simulink model "tailsitter_simulation_main_copy"  (R2021a)
settings: Solver=VariableStepAuto  StartTime=0.0  StopTime=tf  RelTol=1e-3
values from neighbouring files (symbols this model uses):
  b = 0.6    [linear_dynamics_hover.m]    (also in nonlinear_dynamics_eq.m; simulink_setup.m; tailsitter.m; tailsitter_sym.m)
  c_bar = 0.142    [linear_dynamics_hover.m]    (also in nonlinear_dynamics_eq.m; simulink_setup.m; tailsitter.m; tailsitter_sym.m)
  CD_f = 0.000762    [linear_dynamics_hover.m]    (also in nonlinear_dynamics_eq.m; simulink_setup.m; tailsitter.m; tailsitter_sym.m)
  CL_0 = 0    [linear_dynamics_hover.m]    (also in nonlinear_dynamics_eq.m; simulink_setup.m; tailsitter.m; tailsitter_sym.m)
  CL_f = 0.036    [linear_dynamics_hover.m]    (also in nonlinear_dynamics_eq.m; simulink_setup.m; tailsitter.m; tailsitter_sym.m)
  Cl_f = 0.0057    [linear_dynamics_hover.m]    (also in nonlinear_dynamics_eq.m; simulink_setup.m; tailsitter.m; tailsitter_sym.m)
  Cm_0 = 0    [linear_dynamics_hover.m]    (also in nonlinear_dynamics_eq.m; simulink_setup.m; tailsitter.m; tailsitter_sym.m)
  Cm_f = -0.0102    [linear_dynamics_hover.m]    (also in nonlinear_dynamics_eq.m; simulink_setup.m; tailsitter.m; tailsitter_sym.m)
  CP = 0.01    [linear_dynamics_hover.m]    (also in nonlinear_dynamics_eq.m; simulink_setup.m; tailsitter.m; tailsitter_sym.m)
  CT = 0.05    [linear_dynamics_hover.m]    (also in nonlinear_dynamics_eq.m; simulink_setup.m; tailsitter.m; tailsitter_sym.m)
  D = 0.12    [linear_dynamics_hover.m]    (also in nonlinear_dynamics_eq.m; simulink_setup.m; tailsitter.m; tailsitter_sym.m)
  dt = 0.005    [simulink_setup.m]    (also in tailsitter_test.m)
  g = 9.81    [linear_dynamics_hover.m]    (also in nonlinear_dynamics_eq.m; simulink_setup.m; tailsitter.m; tailsitter_sym.m)
  J = [Jxx 0 -Jxz; 0 Jyy 0; -Jxz 0 Jzz]    [linear_dynamics_hover.m]    (also in nonlinear_dynamics_eq.m; simulink_setup.m; tailsitter.m; tailsitter_sym.m)
  Kd = 0.01    [simulink_setup.m]
  Kp = 1    [simulink_setup.m]    (also in tailsitter_test.m = 10)
  Kpi = 10    [simulink_setup.m]    (also in tailsitter_test.m = 100)
  Kq = 1    [simulink_setup.m]    (also in tailsitter_test.m = 10)
  Kqi = 20    [simulink_setup.m]    (also in tailsitter_test.m = 50)
  Kr = 5    [simulink_setup.m]    (also in tailsitter_test.m = 10)
  Kri = 20    [simulink_setup.m]    (also in tailsitter_test.m = 5)
  Kt = -5    [simulink_setup.m]    (also in tailsitter_test.m)
  Kti = -100    [simulink_setup.m]    (also in tailsitter_test.m)
  m = 0.3    [linear_dynamics_hover.m]    (also in nonlinear_dynamics_eq.m; simulink_setup.m; tailsitter.m; tailsitter_sym.m)
  M_flap = [-1 1; -1 -1]    [simulink_setup.m]    (also in tailsitter_test.m)
  M_motor = [1 1; 1 -1]    [simulink_setup.m]    (also in tailsitter_test.m)
  motor_eq = xeq(end)    [simulink_setup.m]
  prop_arm = 0.15    [linear_dynamics_hover.m]    (also in nonlinear_dynamics_eq.m; simulink_setup.m; tailsitter.m; tailsitter_sym.m)
  rho = 1.225    [linear_dynamics_hover.m]    (also in nonlinear_dynamics_eq.m; simulink_setup.m; tailsitter.m; tailsitter_sym.m)
  S_w = S_w/3    (= 0.0276)    [linear_dynamics_hover.m]    (also in nonlinear_dynamics_eq.m; simulink_setup.m = 0.0828; tailsitter.m = 0.0828; tailsitter_sym.m)
libraries: sharedtransform x6, pid_lib x4, vrlib x3, simulink x2, aerolibutil x2, simulink_extras x1, sharedutil x1
settings Model: PacingRate=0.032000  Creator=Owner  LastModifiedBy=Owner

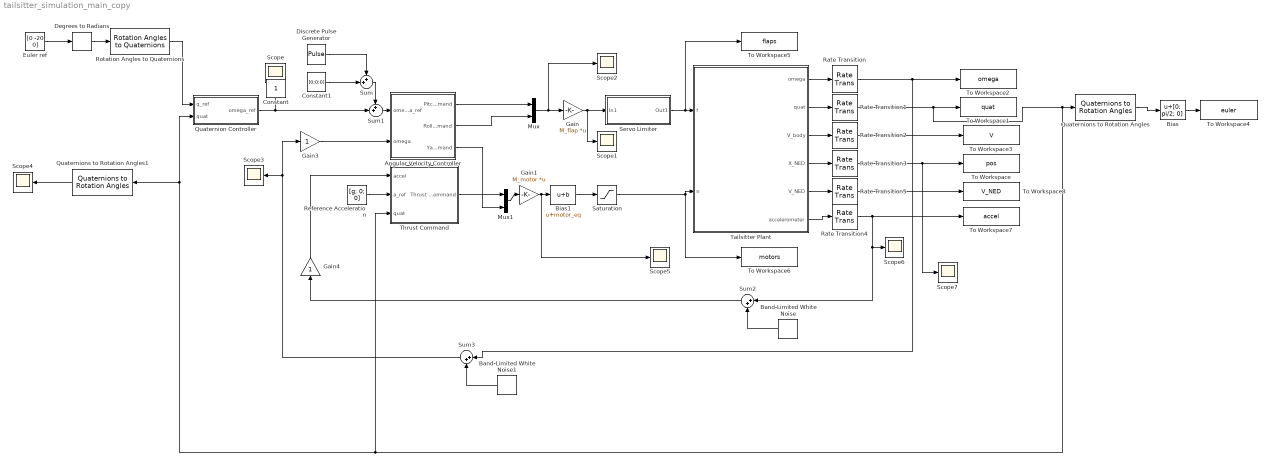
== system tailsitter_simulation_main_copy ==
  Angular Velocity Controller : Subsystem
  Band-Limited White Noise : simulink/Sources/Band-Limited White Noise  Cov=0.01  Ts=dt  seed=[23341]
  Band-Limited White Noise1 : simulink/Sources/Band-Limited White Noise  Cov=0.0001  Ts=dt  seed=[23341]
  Bias : Bias  Bias=[0; pi/2; 0]
  Bias1 : Bias  Bias=motor_eq
  Constant1 : Constant  Value=[0;0;0]  SampleTime=dt
  Degrees to Radians : simulink_extras/Transformations/Degrees to Radians
  Discrete Pulse Generator : DiscretePulseGenerator  Amplitude=0  Period=100000  PulseWidth=20  PhaseDelay=100  SampleTime=dt
  Euler ref : Constant  Value=[0 -20 0]  SampleTime=dt
  Gain : Gain  Gain=M_flap  Multiplication=Matrix(K*u)
  Gain1 : Gain  Gain=M_motor  Multiplication=Matrix(K*u)
  Gain3 : Gain
  Gain4 : Gain
  Mux : Mux  Inputs=2
  Mux1 : Mux  Inputs=2
  Quaternion Controller : Subsystem
  Quaternions to Rotation Angles : sharedtransform/Quaternions to Rotation Angles  rotationOrder=ZYX  aMode=aMode
      settings: SourceProductBaseCode=AE,PW,DR,MT,UV,VE
  Quaternions to Rotation Angles1 : sharedtransform/Quaternions to Rotation Angles  rotationOrder=ZYX  aMode=aMode
      settings: SourceProductBaseCode=AE,PW,DR,MT,UV,VE
  Rate Transition{,1..3,5} (5 alike) : RateTransition  OutPortSampleTime=dt
  Rate Transition4 : RateTransition  OutPortSampleTime=0.005
  Reference Acceleration : Constant  Value=[g; 0; 0]  SampleTime=dt
  Rotation Angles to Quaternions : sharedtransform/Rotation Angles to Quaternions  rotationOrder=ZYX  aMode=aMode
      settings: SourceProductBaseCode=AE,PW,DR,MT,UV,VE
  Saturation : Saturate  UpperLimit=500  LowerLimit=0
  Scope{,1..7} (8 alike) : Scope
  Servo Limiter : Subsystem
  Sum : Sum  Inputs=++|
  Sum1 : Sum  Inputs=++|
  Sum2 : Sum  Inputs=|++
  Sum3 : Sum  Inputs=|++
  Tailsitter Plant : Subsystem
  Thrust Command : Subsystem
  To Workspace : ToWorkspace  VariableName=pos  SampleTime=-1
  To Workspace1 : ToWorkspace  VariableName=quat  SampleTime=-1
  To Workspace2 : ToWorkspace  VariableName=omega  SampleTime=-1
  To Workspace3 : ToWorkspace  VariableName=V  SampleTime=-1
  To Workspace4 : ToWorkspace  VariableName=euler  SampleTime=-1
  To Workspace5 : ToWorkspace  VariableName=flaps  SampleTime=-1
  To Workspace6 : ToWorkspace  VariableName=motors  SampleTime=-1
  To Workspace7 : ToWorkspace  VariableName=accel  SampleTime=-1
  To Workspace8 : ToWorkspace  VariableName=V_NED  SampleTime=-1
  Constant : Constant  IOType=siggen
  wires:
  Tailsitter Plant/4(X_NED) -> Rate Transition3/1
  Tailsitter Plant/1(omega) -> Rate Transition/1
  Tailsitter Plant/2(quat) -> Rate Transition1/1
  Tailsitter Plant/3(V_body) -> Rate Transition2/1
  Quaternions to Rotation Angles/1 -> Bias/1
  Bias/1 -> To Workspace4/1
  Gain1/1 -> Scope5/1, Bias1/1
  Gain/1 -> Scope1/1, Servo Limiter/1(In1)
  Angular Velocity Controller/1(Pitch Command) -> Mux/1
  Angular Velocity Controller/2(Roll Command) -> Mux/2
  Mux/1 -> Scope2/1, Gain/1
  Angular Velocity Controller/3(Yaw Command) -> Mux1/2
  Mux1/1 -> Gain1/1
  Thrust Command/1(Thrust Command) -> Mux1/1
  Tailsitter Plant/6(accelerometer) -> Rate Transition4/1
  Reference Acceleration/1 -> Thrust Command/2(a_ref)
  Rotation Angles to Quaternions/1 -> Quaternion Controller/1(q_ref)
  Degrees to Radians/1 -> Rotation Angles to Quaternions/1
  Euler ref/1 -> Degrees to Radians/1
  Rate Transition/1 -> Sum3/1, To Workspace2/1
  Rate Transition2/1 -> To Workspace3/1
  Rate Transition3/1 -> Scope7/1, To Workspace/1
  Rate Transition4/1 -> Sum2/1, Scope6/1, To Workspace7/1
  Bias1/1 -> Saturation/1
  Servo Limiter/1(Out1) -> To Workspace5/1, Tailsitter Plant/1(f)
  Saturation/1 -> Tailsitter Plant/2(n), To Workspace6/1
  Quaternions to Rotation Angles1/1 -> Scope4/1
  Rate Transition1/1 -> Quaternion Controller/2(quat), Quaternions to Rotation Angles1/1, Thrust Command/3(quat), Quaternions to Rotation Angles/1, To Workspace1/1
  Gain3/1 -> Angular Velocity Controller/2(omega)
  Gain4/1 -> Thrust Command/1(accel)
  Rate Transition5/1 -> To Workspace8/1
  Tailsitter Plant/5(V_NED) -> Rate Transition5/1
  Discrete Pulse Generator/1 -> Sum/1
  Constant1/1 -> Sum/2
  Sum/1 -> Sum1/1
  Sum1/1 -> Angular Velocity Controller/1(omega_ref)
  Quaternion Controller/1(omega_ref) -> Sum1/2, Scope/1
  Band-Limited White Noise/1 -> Sum2/2
  Sum2/1 -> Gain4/1
  Band-Limited White Noise1/1 -> Sum3/2
  Sum3/1 -> Gain3/1, Scope3/1

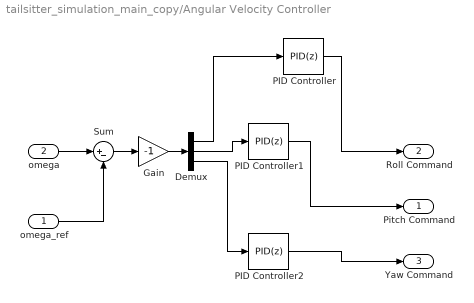
== system tailsitter_simulation_main_copy/Angular Velocity Controller ==
  omega_ref : Inport
  omega : Inport  Port=2
  Demux : Demux  Outputs=3
  Gain : Gain  Gain=-1
  PID Controller : pid_lib/PID Controller  Controller=PID  Form=Parallel  TimeDomain=Discrete-time  UseExternalTs=off  SampleTime=-1  IntegratorMethod=Forward Euler  FilterMethod=Forward Euler  ControllerParametersSource=internal  P=Kp  I=Kpi  D=Kd  UseFilter=on  N=100  TunerSelectOption=Transfer Function Based (PID Tuner App)  InitialConditionSource=internal  InitialConditionForIntegrator=0  InitialConditionForFilter=0  DifferentiatorICPrevScaledInput=0  ExternalReset=none  TrackingMode=off  Kt=1  LimitOutput=off  SatLimitsSource=internal  UpperSaturationLimit=inf  LowerSaturationLimit=-inf  LinearizeAsGain=on  AntiWindupMode=none  Kb=1  POutMin=[]  POutMax=[]  IOutMin=[]  IOutMax=[]  DOutMin=[]  DOutMax=[]  NOutMin=[]  NOutMax=[]  SumOutMin=[]  SumOutMax=[]  SaturationOutMin=[]  SaturationOutMax=[]  PParamMin=[]  PParamMax=[]  IParamMin=[]  IParamMax=[]  DParamMin=[]  DParamMax=[]  NParamMin=[]  NParamMax=[]  KbParamMin=[]  KbParamMax=[]  KtParamMin=[]  KtParamMax=[]  KbOutMin=[]  KbOutMax=[]  KtOutMin=[]  KtOutMax=[]  IntegratorOutMin=[]  IntegratorOutMax=[]  FilterOutMin=[]  FilterOutMax=[]  SumI1OutMin=[]  SumI1OutMax=[]  SumI2OutMin=[]  SumI2OutMax=[]  SumI3OutMin=[]  SumI3OutMax=[]  SumI4OutMin=[]  SumI4OutMax=[]  SumDOutMin=[]  SumDOutMax=[]  DifferentiatorOutMin=[]  DifferentiatorOutMax=[]  FilterDiffOutCoefMin=[]  FilterDiffOutCoefMax=[]  ReciprocalOutMin=[]  ReciprocalOutMax=[]  SumDenOutMin=[]  SumDenOutMax=[]  SumNumOutMin=[]  SumNumOutMax=[]  DivideOutMin=[]  DivideOutMax=[]  UdiffTsProdOutMin=[]  UdiffTsProdOutMax=[]  NTsProdOutMin=[]  NTsProdOutMax=[]  UintegralTsProdOutMin=[]  UintegralTsProdOutMax=[]  UngainTsProdOutMin=[]  UngainTsProdOutMax=[]  IntegratorContinuousStateAttributes=''  IntegratorStateMustResolveToSignalObject=off  IntegratorRTWStateStorageClass=Auto  FilterContinuousStateAttributes=''  FilterStateMustResolveToSignalObject=off  FilterRTWStateStorageClass=Auto  ParallelPVariant=InternalParameters  IdealPVariant=Disabled  IVariant=InternalParameters  DVariant=InternalParameters  IntegratorVariant=Discrete  SatVariant=Disabled  AWVariant=Passthrough  PCopyVariant=Disabled  TRVariant=Disabled  FdbkBlocksVariant=Forward  IdealPFdbkVariant=Disabled  SatFdbkVariant=Disabled  DerivativeFilterVariant=ForwardEulerFilter  NVariant=InternalParameters  NCopyVariant=Disabled  FilterICVariant=InternalICsFilter  IntegratorICVariant=InternalICs  ExternalResetVariant=Disabled  TRSumVariant=Passthrough  SumFdbkVariant=Disabled  SumVariant=Sum_PID  TsampFilterVariant=InternalTs  TsampNgainVariant=Passthrough  TsampIntegralVariant=Passthrough  ExternalSaturationOutDataTypeStr=Inherit: Same as second input
  PID Controller1 : pid_lib/PID Controller  Controller=PID  Form=Parallel  TimeDomain=Discrete-time  UseExternalTs=off  SampleTime=-1  IntegratorMethod=Forward Euler  FilterMethod=Forward Euler  ControllerParametersSource=internal  P=Kq  I=Kqi  D=Kd  UseFilter=on  N=100  TunerSelectOption=Transfer Function Based (PID Tuner App)  InitialConditionSource=internal  InitialConditionForIntegrator=0  InitialConditionForFilter=0  DifferentiatorICPrevScaledInput=0  ExternalReset=none  TrackingMode=off  Kt=1  LimitOutput=off  SatLimitsSource=internal  UpperSaturationLimit=inf  LowerSaturationLimit=-inf  LinearizeAsGain=on  AntiWindupMode=none  Kb=1  POutMin=[]  POutMax=[]  IOutMin=[]  IOutMax=[]  DOutMin=[]  DOutMax=[]  NOutMin=[]  NOutMax=[]  SumOutMin=[]  SumOutMax=[]  SaturationOutMin=[]  SaturationOutMax=[]  PParamMin=[]  PParamMax=[]  IParamMin=[]  IParamMax=[]  DParamMin=[]  DParamMax=[]  NParamMin=[]  NParamMax=[]  KbParamMin=[]  KbParamMax=[]  KtParamMin=[]  KtParamMax=[]  KbOutMin=[]  KbOutMax=[]  KtOutMin=[]  KtOutMax=[]  IntegratorOutMin=[]  IntegratorOutMax=[]  FilterOutMin=[]  FilterOutMax=[]  SumI1OutMin=[]  SumI1OutMax=[]  SumI2OutMin=[]  SumI2OutMax=[]  SumI3OutMin=[]  SumI3OutMax=[]  SumI4OutMin=[]  SumI4OutMax=[]  SumDOutMin=[]  SumDOutMax=[]  DifferentiatorOutMin=[]  DifferentiatorOutMax=[]  FilterDiffOutCoefMin=[]  FilterDiffOutCoefMax=[]  ReciprocalOutMin=[]  ReciprocalOutMax=[]  SumDenOutMin=[]  SumDenOutMax=[]  SumNumOutMin=[]  SumNumOutMax=[]  DivideOutMin=[]  DivideOutMax=[]  UdiffTsProdOutMin=[]  UdiffTsProdOutMax=[]  NTsProdOutMin=[]  NTsProdOutMax=[]  UintegralTsProdOutMin=[]  UintegralTsProdOutMax=[]  UngainTsProdOutMin=[]  UngainTsProdOutMax=[]  IntegratorContinuousStateAttributes=''  IntegratorStateMustResolveToSignalObject=off  IntegratorRTWStateStorageClass=Auto  FilterContinuousStateAttributes=''  FilterStateMustResolveToSignalObject=off  FilterRTWStateStorageClass=Auto  ParallelPVariant=InternalParameters  IdealPVariant=Disabled  IVariant=InternalParameters  DVariant=InternalParameters  IntegratorVariant=Discrete  SatVariant=Disabled  AWVariant=Passthrough  PCopyVariant=Disabled  TRVariant=Disabled  FdbkBlocksVariant=Forward  IdealPFdbkVariant=Disabled  SatFdbkVariant=Disabled  DerivativeFilterVariant=ForwardEulerFilter  NVariant=InternalParameters  NCopyVariant=Disabled  FilterICVariant=InternalICsFilter  IntegratorICVariant=InternalICs  ExternalResetVariant=Disabled  TRSumVariant=Passthrough  SumFdbkVariant=Disabled  SumVariant=Sum_PID  TsampFilterVariant=InternalTs  TsampNgainVariant=Passthrough  TsampIntegralVariant=Passthrough  ExternalSaturationOutDataTypeStr=Inherit: Same as second input
  PID Controller2 : pid_lib/PID Controller  Controller=PID  Form=Parallel  TimeDomain=Discrete-time  UseExternalTs=off  SampleTime=-1  IntegratorMethod=Forward Euler  FilterMethod=Forward Euler  ControllerParametersSource=internal  P=Kr*5  I=Kri  D=Kd*100  UseFilter=on  N=100  TunerSelectOption=Transfer Function Based (PID Tuner App)  InitialConditionSource=internal  InitialConditionForIntegrator=0  InitialConditionForFilter=0  DifferentiatorICPrevScaledInput=0  ExternalReset=none  TrackingMode=off  Kt=1  LimitOutput=off  SatLimitsSource=internal  UpperSaturationLimit=inf  LowerSaturationLimit=-inf  LinearizeAsGain=on  AntiWindupMode=none  Kb=1  POutMin=[]  POutMax=[]  IOutMin=[]  IOutMax=[]  DOutMin=[]  DOutMax=[]  NOutMin=[]  NOutMax=[]  SumOutMin=[]  SumOutMax=[]  SaturationOutMin=[]  SaturationOutMax=[]  PParamMin=[]  PParamMax=[]  IParamMin=[]  IParamMax=[]  DParamMin=[]  DParamMax=[]  NParamMin=[]  NParamMax=[]  KbParamMin=[]  KbParamMax=[]  KtParamMin=[]  KtParamMax=[]  KbOutMin=[]  KbOutMax=[]  KtOutMin=[]  KtOutMax=[]  IntegratorOutMin=[]  IntegratorOutMax=[]  FilterOutMin=[]  FilterOutMax=[]  SumI1OutMin=[]  SumI1OutMax=[]  SumI2OutMin=[]  SumI2OutMax=[]  SumI3OutMin=[]  SumI3OutMax=[]  SumI4OutMin=[]  SumI4OutMax=[]  SumDOutMin=[]  SumDOutMax=[]  DifferentiatorOutMin=[]  DifferentiatorOutMax=[]  FilterDiffOutCoefMin=[]  FilterDiffOutCoefMax=[]  ReciprocalOutMin=[]  ReciprocalOutMax=[]  SumDenOutMin=[]  SumDenOutMax=[]  SumNumOutMin=[]  SumNumOutMax=[]  DivideOutMin=[]  DivideOutMax=[]  UdiffTsProdOutMin=[]  UdiffTsProdOutMax=[]  NTsProdOutMin=[]  NTsProdOutMax=[]  UintegralTsProdOutMin=[]  UintegralTsProdOutMax=[]  UngainTsProdOutMin=[]  UngainTsProdOutMax=[]  IntegratorContinuousStateAttributes=''  IntegratorStateMustResolveToSignalObject=off  IntegratorRTWStateStorageClass=Auto  FilterContinuousStateAttributes=''  FilterStateMustResolveToSignalObject=off  FilterRTWStateStorageClass=Auto  ParallelPVariant=InternalParameters  IdealPVariant=Disabled  IVariant=InternalParameters  DVariant=InternalParameters  IntegratorVariant=Discrete  SatVariant=Disabled  AWVariant=Passthrough  PCopyVariant=Disabled  TRVariant=Disabled  FdbkBlocksVariant=Forward  IdealPFdbkVariant=Disabled  SatFdbkVariant=Disabled  DerivativeFilterVariant=ForwardEulerFilter  NVariant=InternalParameters  NCopyVariant=Disabled  FilterICVariant=InternalICsFilter  IntegratorICVariant=InternalICs  ExternalResetVariant=Disabled  TRSumVariant=Passthrough  SumFdbkVariant=Disabled  SumVariant=Sum_PID  TsampFilterVariant=InternalTs  TsampNgainVariant=Passthrough  TsampIntegralVariant=Passthrough  ExternalSaturationOutDataTypeStr=Inherit: Same as second input
  Sum : Sum  Inputs=|+-
  Pitch Command : Outport
  Roll Command : Outport  Port=2
  Yaw Command : Outport  Port=3
  wires:
  omega_ref/1 -> Sum/2
  omega/1 -> Sum/1
  Sum/1 -> Gain/1
  Demux/2 -> PID Controller1/1
  Demux/3 -> PID Controller2/1
  Demux/1 -> PID Controller/1
  PID Controller2/1 -> Yaw Command/1
  PID Controller1/1 -> Pitch Command/1
  PID Controller/1 -> Roll Command/1
  Gain/1 -> Demux/1

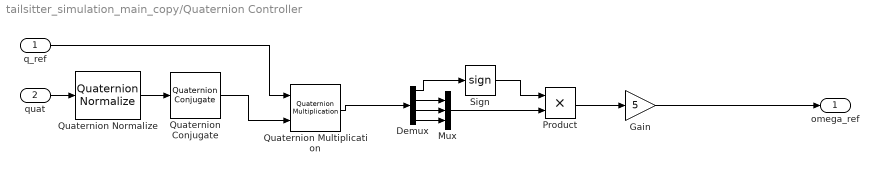
== system tailsitter_simulation_main_copy/Quaternion Controller ==
  q_ref : Inport
  quat : Inport  Port=2
  Demux : Demux
  Gain : Gain  Gain=5
  Mux : Mux  Inputs=3
  Product : Product
  Quaternion Conjugate : aerolibutil/Quaternion Conjugate
      settings: SourceProductBaseCode=AE
  Quaternion Multiplication : aerolibutil/Quaternion Multiplication
  Quaternion Normalize : sharedutil/Quaternion Normalize  aMode=aMode
      settings: SourceProductBaseCode=AE,PW,DR,MT,UV,VE
  Sign : Signum
  omega_ref : Outport
  wires:
  quat/1 -> Quaternion Normalize/1
  q_ref/1 -> Quaternion Multiplication/1
  Quaternion Multiplication/1 -> Demux/1
  Product/1 -> Gain/1
  Demux/1 -> Sign/1
  Sign/1 -> Product/1
  Demux/2 -> Mux/1
  Demux/3 -> Mux/2
  Demux/4 -> Mux/3
  Mux/1 -> Product/2
  Quaternion Conjugate/1 -> Quaternion Multiplication/2
  Gain/1 -> omega_ref/1
  Quaternion Normalize/1 -> Quaternion Conjugate/1

== system tailsitter_simulation_main_copy/Servo Limiter ==
  In1 : Inport
  Rate Limiter : RateLimiter  RisingSlewLimit=400  FallingSlewLimit=-400  SampleTimeMode=inherited
  Saturation : Saturate  UpperLimit=20  LowerLimit=-20
  Out1 : Outport
  wires:
  In1/1 -> Saturation/1
  Saturation/1 -> Rate Limiter/1
  Rate Limiter/1 -> Out1/1

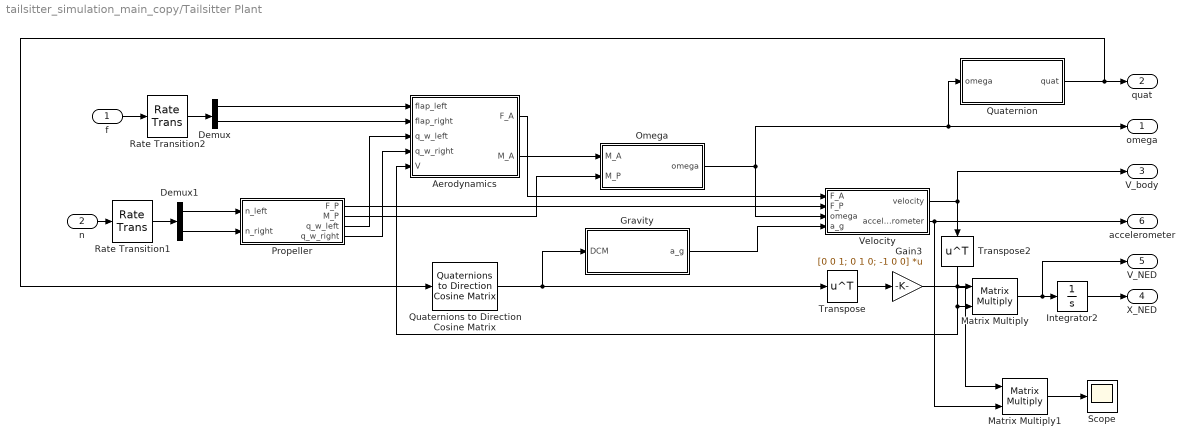
== system tailsitter_simulation_main_copy/Tailsitter Plant ==
  f : Inport
  n : Inport  Port=2
  Aerodynamics : Subsystem
  Demux : Demux  Outputs=2
  Demux1 : Demux  Outputs=2
  Gain3 : Gain  Gain=[0 0 1; 0 1 0; -1 0 0]  Multiplication=Matrix(K*u)
  Gravity : Subsystem
  Integrator2 : Integrator  InitialCondition=[0;0;-2]
  Matrix Multiply : Product  Multiplication=Matrix(*)
  Matrix Multiply1 : Product  Multiplication=Matrix(*)
  Omega : Subsystem
  Propeller : Subsystem
  Quaternion : Subsystem
  Quaternions to Direction Cosine Matrix : sharedtransform/Quaternions to  Direction Cosine Matrix  aMode=aMode
      settings: SourceProductBaseCode=AE,PW,DR,MT,UV,VE
  Rate Transition1 : RateTransition  OutPortSampleTimeOpt=Inherit
  Rate Transition2 : RateTransition  OutPortSampleTimeOpt=Inherit
  Scope : Scope
  Transpose : Math  Operator=transpose  SaturateOnIntegerOverflow=on
  Transpose2 : Math  Operator=transpose  SaturateOnIntegerOverflow=on
  Velocity : Subsystem
  omega : Outport
  quat : Outport  Port=2
  V_body : Outport  Port=3
  X_NED : Outport  Port=4
  V_NED : Outport  Port=5
  accelerometer : Outport  Port=6
  wires:
  Aerodynamics/1(F_A) -> Velocity/1(F_A)
  Demux/1 -> Aerodynamics/1(flap_left)
  Demux/2 -> Aerodynamics/2(flap_right)
  Demux1/1 -> Propeller/1(n_left)
  Demux1/2 -> Propeller/2(n_right)
  Propeller/2(M_P) -> Omega/2(M_P)
  Quaternions to Direction Cosine Matrix/1 -> Transpose/1, Gravity/1(DCM)
  Gain3/1 -> Matrix Multiply1/1, Matrix Multiply/1
  Transpose/1 -> Gain3/1
  Matrix Multiply/1 -> V_NED/1, Integrator2/1
  Integrator2/1 -> X_NED/1
  n/1 -> Rate Transition1/1
  Omega/1(omega) -> Quaternion/1(omega), omega/1, Velocity/3(omega)
  Aerodynamics/2(M_A) -> Omega/1(M_A)
  Velocity/1(velocity) -> V_body/1, Transpose2/1
  Velocity/2(accelerometer) -> accelerometer/1, Matrix Multiply1/2
  Gravity/1(a_g) -> Velocity/4(a_g)
  Propeller/1(F_P) -> Velocity/2(F_P)
  Quaternion/1(quat) -> Quaternions to Direction Cosine Matrix/1, quat/1
  Transpose2/1 -> Aerodynamics/5(V), Matrix Multiply/2
  f/1 -> Rate Transition2/1
  Rate Transition1/1 -> Demux1/1
  Propeller/3(q_w_left) -> Aerodynamics/3(q_w_left)
  Propeller/4(q_w_right) -> Aerodynamics/4(q_w_right)
  Rate Transition2/1 -> Demux/1
  Matrix Multiply1/1 -> Scope/1

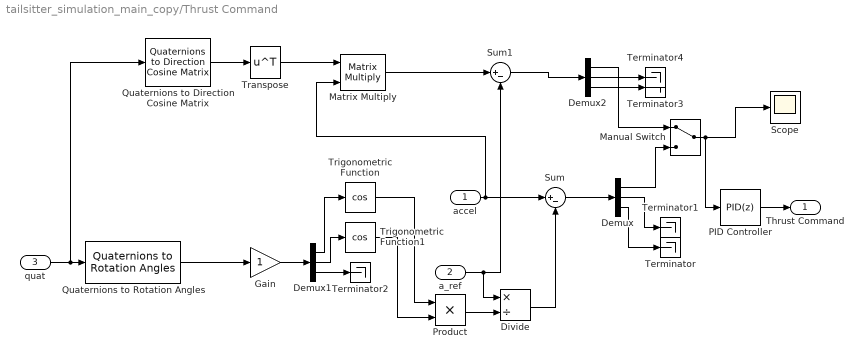
== system tailsitter_simulation_main_copy/Thrust Command ==
  accel : Inport
  a_ref : Inport  Port=2
  quat : Inport  Port=3
  Demux : Demux  Outputs=3
  Demux1 : Demux  Outputs=3
  Demux2 : Demux  Outputs=3
  Divide : Product  Inputs=*/
  Gain : Gain
  Manual Switch : ManualSwitch
  Matrix Multiply : Product  Multiplication=Matrix(*)
  PID Controller : pid_lib/PID Controller  Controller=PID  Form=Parallel  TimeDomain=Discrete-time  UseExternalTs=off  SampleTime=-1  IntegratorMethod=Forward Euler  FilterMethod=Forward Euler  ControllerParametersSource=internal  P=Kt  I=Kti  D=0  UseFilter=on  N=100  TunerSelectOption=Transfer Function Based (PID Tuner App)  InitialConditionSource=internal  InitialConditionForIntegrator=0  InitialConditionForFilter=0  DifferentiatorICPrevScaledInput=0  ExternalReset=none  TrackingMode=off  Kt=1  LimitOutput=off  SatLimitsSource=internal  UpperSaturationLimit=inf  LowerSaturationLimit=-inf  LinearizeAsGain=on  AntiWindupMode=none  Kb=1  POutMin=[]  POutMax=[]  IOutMin=[]  IOutMax=[]  DOutMin=[]  DOutMax=[]  NOutMin=[]  NOutMax=[]  SumOutMin=[]  SumOutMax=[]  SaturationOutMin=[]  SaturationOutMax=[]  PParamMin=[]  PParamMax=[]  IParamMin=[]  IParamMax=[]  DParamMin=[]  DParamMax=[]  NParamMin=[]  NParamMax=[]  KbParamMin=[]  KbParamMax=[]  KtParamMin=[]  KtParamMax=[]  KbOutMin=[]  KbOutMax=[]  KtOutMin=[]  KtOutMax=[]  IntegratorOutMin=[]  IntegratorOutMax=[]  FilterOutMin=[]  FilterOutMax=[]  SumI1OutMin=[]  SumI1OutMax=[]  SumI2OutMin=[]  SumI2OutMax=[]  SumI3OutMin=[]  SumI3OutMax=[]  SumI4OutMin=[]  SumI4OutMax=[]  SumDOutMin=[]  SumDOutMax=[]  DifferentiatorOutMin=[]  DifferentiatorOutMax=[]  FilterDiffOutCoefMin=[]  FilterDiffOutCoefMax=[]  ReciprocalOutMin=[]  ReciprocalOutMax=[]  SumDenOutMin=[]  SumDenOutMax=[]  SumNumOutMin=[]  SumNumOutMax=[]  DivideOutMin=[]  DivideOutMax=[]  UdiffTsProdOutMin=[]  UdiffTsProdOutMax=[]  NTsProdOutMin=[]  NTsProdOutMax=[]  UintegralTsProdOutMin=[]  UintegralTsProdOutMax=[]  UngainTsProdOutMin=[]  UngainTsProdOutMax=[]  IntegratorContinuousStateAttributes=''  IntegratorStateMustResolveToSignalObject=off  IntegratorRTWStateStorageClass=Auto  FilterContinuousStateAttributes=''  FilterStateMustResolveToSignalObject=off  FilterRTWStateStorageClass=Auto  ParallelPVariant=InternalParameters  IdealPVariant=Disabled  IVariant=InternalParameters  DVariant=InternalParameters  IntegratorVariant=Discrete  SatVariant=Disabled  AWVariant=Passthrough  PCopyVariant=Disabled  TRVariant=Disabled  FdbkBlocksVariant=Forward  IdealPFdbkVariant=Disabled  SatFdbkVariant=Disabled  DerivativeFilterVariant=ForwardEulerFilter  NVariant=InternalParameters  NCopyVariant=Disabled  FilterICVariant=InternalICsFilter  IntegratorICVariant=InternalICs  ExternalResetVariant=Disabled  TRSumVariant=Passthrough  SumFdbkVariant=Disabled  SumVariant=Sum_PID  TsampFilterVariant=InternalTs  TsampNgainVariant=Passthrough  TsampIntegralVariant=Passthrough  ExternalSaturationOutDataTypeStr=Inherit: Same as second input
  Product : Product
  Quaternions to Direction Cosine Matrix : sharedtransform/Quaternions to  Direction Cosine Matrix  aMode=aMode
      settings: SourceProductBaseCode=AE,PW,DR,MT,UV,VE
  Quaternions to Rotation Angles : sharedtransform/Quaternions to Rotation Angles  rotationOrder=ZYX  aMode=aMode
      settings: SourceProductBaseCode=AE,PW,DR,MT,UV,VE
  Scope : Scope
  Sum : Sum  Inputs=|+-
  Sum1 : Sum  Inputs=|+-
  Terminator{,1..4} (5 alike) : Terminator
  Transpose : Math  Operator=transpose  SaturateOnIntegerOverflow=on
  Trigonometric Function : Trigonometry  Operator=cos
  Trigonometric Function1 : Trigonometry  Operator=cos
  Thrust Command : Outport
  wires:
  quat/1 -> Quaternions to Direction Cosine Matrix/1, Quaternions to Rotation Angles/1
  accel/1 -> Matrix Multiply/2, Sum/1
  Sum/1 -> Demux/1
  a_ref/1 -> Sum1/2, Divide/1
  Divide/1 -> Sum/2
  Demux/3 -> Terminator/1
  Demux/2 -> Terminator1/1
  PID Controller/1 -> Thrust Command/1
  Quaternions to Rotation Angles/1 -> Gain/1
  Demux1/3 -> Terminator2/1
  Demux1/1 -> Trigonometric Function/1
  Demux1/2 -> Trigonometric Function1/1
  Quaternions to Direction Cosine Matrix/1 -> Transpose/1
  Trigonometric Function/1 -> Product/1
  Product/1 -> Divide/2
  Trigonometric Function1/1 -> Product/2
  Gain/1 -> Demux1/1
  Demux/1 -> Manual Switch/2
  Transpose/1 -> Matrix Multiply/1
  Matrix Multiply/1 -> Sum1/1
  Sum1/1 -> Demux2/1
  Demux2/2 -> Terminator4/1
  Demux2/3 -> Terminator3/1
  Manual Switch/1 -> PID Controller/1, Scope/1
  Demux2/1 -> Manual Switch/1

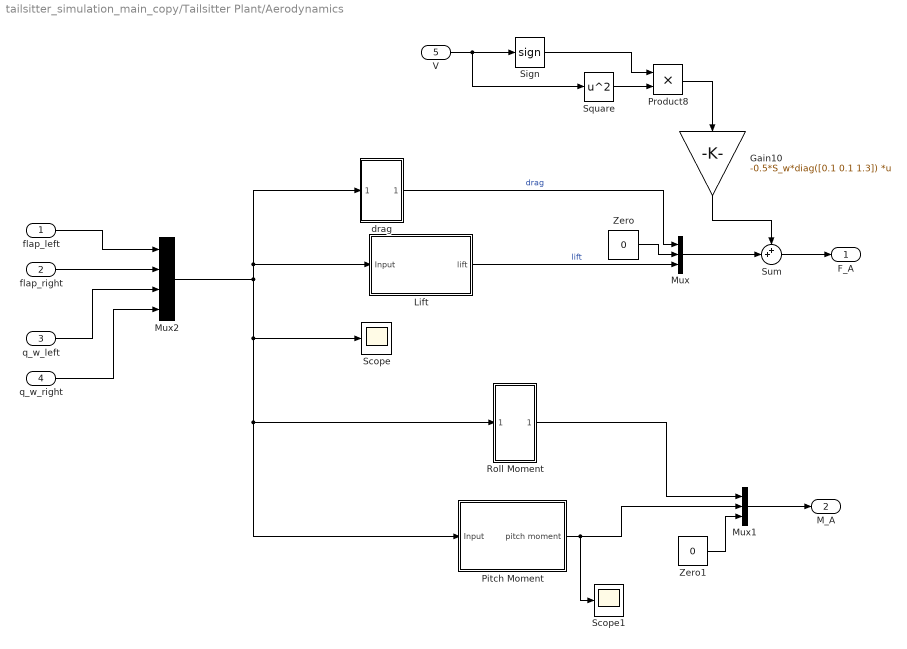
== system tailsitter_simulation_main_copy/Tailsitter Plant/Aerodynamics ==
  flap_left : Inport
  flap_right : Inport  Port=2
  q_w_left : Inport  Port=3
  q_w_right : Inport  Port=4
  V : Inport  Port=5
  Gain10 : Gain  Gain=-0.5*S_w*diag([0.1 0.1 1.3])  Multiplication=Matrix(K*u) (u vector)
  Lift : Subsystem
  Mux : Mux  Inputs=3
  Mux1 : Mux  Inputs=3
  Mux2 : Mux
  Pitch Moment : Subsystem
  Product8 : Product
  Roll Moment : Subsystem
  Scope : Scope
  Scope1 : Scope
  Sign : Signum
  Square : Math  Operator=square  SaturateOnIntegerOverflow=on
  Sum : Sum  Inputs=++|
  Zero : Constant  Value=0  OutDataTypeStr=Inherit: Inherit via back propagation
  Zero1 : Constant  Value=0  OutDataTypeStr=Inherit: Inherit via back propagation
  drag : Subsystem
  F_A : Outport
  M_A : Outport  Port=2
  wires:
  Lift/1(lift) -> Mux/3  "lift"
  Zero/1 -> Mux/2
  drag/1(drag) -> Mux/1  "drag"
  flap_left/1 -> Mux2/1
  flap_right/1 -> Mux2/2
  Mux1/1 -> M_A/1
  Zero1/1 -> Mux1/3
  V/1 -> Sign/1, Square/1
  Square/1 -> Product8/2
  Sign/1 -> Product8/1
  Product8/1 -> Gain10/1
  Gain10/1 -> Sum/1
  q_w_right/1 -> Mux2/4
  q_w_left/1 -> Mux2/3
  Pitch Moment/1(pitch moment) -> Scope1/1, Mux1/2
  Roll Moment/1(Out1) -> Mux1/1
  Mux2/1 -> Pitch Moment/1(Input), Roll Moment/1(Input), Scope/1, drag/1(Input), Lift/1(Input)
  Mux/1 -> Sum/2
  Sum/1 -> F_A/1

== system tailsitter_simulation_main_copy/Tailsitter Plant/Gravity ==
  DCM : Inport
  Constant : Constant  Value=-g
  Matrix Multiply : Product  Multiplication=Matrix(*)
  Mux : Mux  Inputs=3
  Zero : Constant  Value=0  OutDataTypeStr=Inherit: Inherit via back propagation
  a_g : Outport
  wires:
  Mux/1 -> Matrix Multiply/2
  Constant/1 -> Mux/1
  Zero/1 -> Mux/3, Mux/2
  Matrix Multiply/1 -> a_g/1
  DCM/1 -> Matrix Multiply/1

== system tailsitter_simulation_main_copy/Tailsitter Plant/Omega ==
  M_A : Inport
  M_P : Inport  Port=2
  Cross Product1 : vrlib/Utilities/Cross Product
  Gain : Gain  Gain=inv(J)  Multiplication=Matrix(K*u) (u vector)
  Gain1 : Gain  Gain=J  Multiplication=Matrix(K*u) (u vector)
  Integrator1 : Integrator
  Sum : Sum  Inputs=|-++
  omega : Outport
  wires:
  Sum/1 -> Gain/1
  Cross Product1/1 -> Sum/1
  M_P/1 -> Sum/2
  Integrator1/1 -> omega/1, Cross Product1/1, Gain1/1
  Gain1/1 -> Cross Product1/2
  Gain/1 -> Integrator1/1
  M_A/1 -> Sum/3

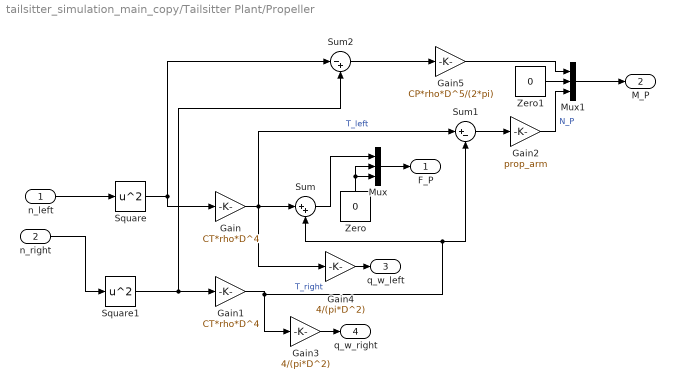
== system tailsitter_simulation_main_copy/Tailsitter Plant/Propeller ==
  n_left : Inport
  n_right : Inport  Port=2
  Gain : Gain  Gain=CT*rho*D^4
  Gain1 : Gain  Gain=CT*rho*D^4
  Gain2 : Gain  Gain=prop_arm
  Gain3 : Gain  Gain=4/(pi*D^2)
  Gain4 : Gain  Gain=4/(pi*D^2)
  Gain5 : Gain  Gain=CP*rho*D^5/(2*pi)
  Mux : Mux  Inputs=3
  Mux1 : Mux  Inputs=3
  Square : Math  Operator=square  SaturateOnIntegerOverflow=on
  Square1 : Math  Operator=square  SaturateOnIntegerOverflow=on
  Sum : Sum  Inputs=|++
  Sum1 : Sum  Inputs=|+-
  Sum2 : Sum  Inputs=|-+
  Zero : Constant  Value=0  OutDataTypeStr=Inherit: Inherit via back propagation
  Zero1 : Constant  Value=0  OutDataTypeStr=Inherit: Inherit via back propagation
  F_P : Outport
  M_P : Outport  Port=2
  q_w_left : Outport  Port=3
  q_w_right : Outport  Port=4
  wires:
  Gain/1 -> Sum1/1, Gain4/1, Sum/1  "T_left"
  Gain1/1 -> Gain3/1, Sum/2, Sum1/2  "T_right"
  n_right/1 -> Square1/1
  Gain3/1 -> q_w_right/1
  n_left/1 -> Square/1
  Gain4/1 -> q_w_left/1
  Mux/1 -> F_P/1
  Sum/1 -> Mux/1
  Zero/1 -> Mux/3, Mux/2
  Mux1/1 -> M_P/1
  Zero1/1 -> Mux1/2
  Gain2/1 -> Mux1/3  "N_P"
  Sum1/1 -> Gain2/1
  Gain5/1 -> Mux1/1
  Square/1 -> Gain/1, Sum2/1
  Square1/1 -> Sum2/2, Gain1/1
  Sum2/1 -> Gain5/1

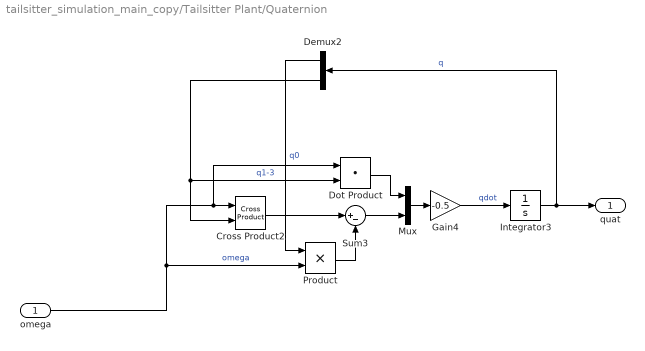
== system tailsitter_simulation_main_copy/Tailsitter Plant/Quaternion ==
  omega : Inport
  Cross Product2 : vrlib/Utilities/Cross Product
  Demux2 : Demux  Outputs=2
  Dot Product : DotProduct  InputSameDT=on  OutDataTypeStr=Inherit: Inherit via internal rule
  Gain4 : Gain  Gain=-0.5
  Integrator3 : Integrator  InitialCondition=[1; 0; 0; 0]
  Mux : Mux  Inputs=2
  Product : Product
  Sum3 : Sum  Inputs=|+-
  quat : Outport
  wires:
  Integrator3/1 -> quat/1, Demux2/1  "q"
  Demux2/1 -> Product/1  "q0"
  omega/1 -> Product/2, Cross Product2/1, Dot Product/1  "omega"
  Dot Product/1 -> Mux/1
  Gain4/1 -> Integrator3/1  "qdot"
  Sum3/1 -> Mux/2
  Demux2/2 -> Cross Product2/2, Dot Product/2  "q1-3"
  Mux/1 -> Gain4/1
  Cross Product2/1 -> Sum3/1
  Product/1 -> Sum3/2

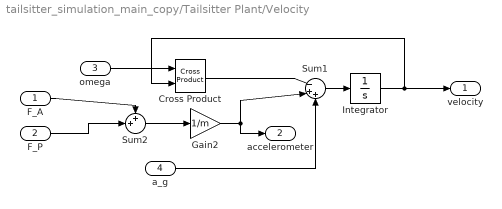
== system tailsitter_simulation_main_copy/Tailsitter Plant/Velocity ==
  F_A : Inport
  F_P : Inport  Port=2
  omega : Inport  Port=3
  a_g : Inport  Port=4
  Cross Product : vrlib/Utilities/Cross Product
  Gain2 : Gain  Gain=1/m
  Integrator : Integrator
  Sum1 : Sum  Inputs=|-++
  Sum2 : Sum  Inputs=++|
  velocity : Outport
  accelerometer : Outport  Port=2
  wires:
  Sum2/1 -> Gain2/1
  F_A/1 -> Sum2/1
  Gain2/1 -> accelerometer/1, Sum1/2
  a_g/1 -> Sum1/3
  Sum1/1 -> Integrator/1
  F_P/1 -> Sum2/2
  omega/1 -> Cross Product/1
  Cross Product/1 -> Sum1/1
  Integrator/1 -> Cross Product/2, velocity/1

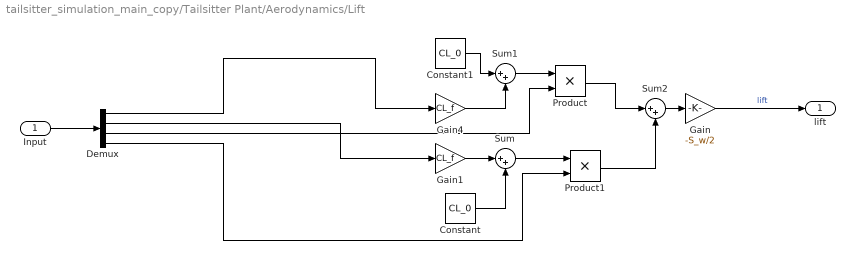
== system tailsitter_simulation_main_copy/Tailsitter Plant/Aerodynamics/Lift ==
  Input : Inport
  Constant : Constant  Value=CL_0
  Constant1 : Constant  Value=CL_0
  Demux : Demux
  Gain : Gain  Gain=-S_w/2
  Gain1 : Gain  Gain=CL_f
  Gain4 : Gain  Gain=CL_f
  Product : Product
  Product1 : Product
  Sum : Sum  Inputs=|++
  Sum1 : Sum  Inputs=|++
  Sum2 : Sum  Inputs=|++
  lift : Outport
  wires:
  Gain1/1 -> Sum/1
  Sum1/1 -> Product/1
  Gain4/1 -> Sum1/2
  Demux/2 -> Gain1/1
  Sum2/1 -> Gain/1
  Product1/1 -> Sum2/2
  Demux/4 -> Product1/2
  Constant1/1 -> Sum1/1
  Sum/1 -> Product1/1
  Demux/3 -> Product/2
  Product/1 -> Sum2/1
  Demux/1 -> Gain4/1
  Constant/1 -> Sum/2
  Gain/1 -> lift/1  "lift"
  Input/1 -> Demux/1

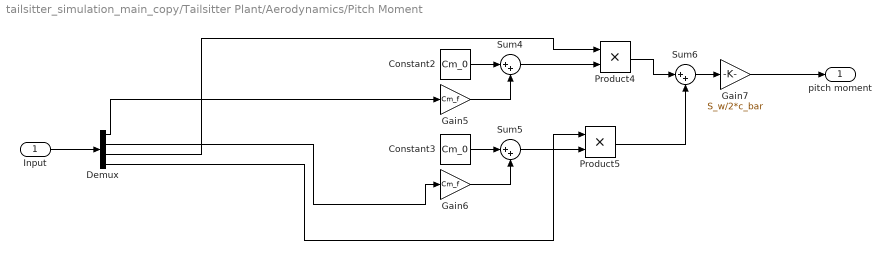
== system tailsitter_simulation_main_copy/Tailsitter Plant/Aerodynamics/Pitch Moment ==
  Input : Inport
  Constant2 : Constant  Value=Cm_0
  Constant3 : Constant  Value=Cm_0
  Demux : Demux
  Gain5 : Gain  Gain=Cm_f
  Gain6 : Gain  Gain=Cm_f
  Gain7 : Gain  Gain=S_w/2*c_bar
  Product4 : Product
  Product5 : Product
  Sum4 : Sum  Inputs=|++
  Sum5 : Sum  Inputs=|++
  Sum6 : Sum  Inputs=|++
  pitch moment : Outport
  wires:
  Constant3/1 -> Sum5/1
  Gain5/1 -> Sum4/2
  Sum4/1 -> Product4/2
  Sum5/1 -> Product5/2
  Gain6/1 -> Sum5/2
  Product4/1 -> Sum6/1
  Sum6/1 -> Gain7/1
  Constant2/1 -> Sum4/1
  Demux/4 -> Product5/1
  Product5/1 -> Sum6/2
  Gain7/1 -> pitch moment/1
  Demux/3 -> Product4/1
  Input/1 -> Demux/1
  Demux/2 -> Gain6/1
  Demux/1 -> Gain5/1

== system tailsitter_simulation_main_copy/Tailsitter Plant/Aerodynamics/Roll Moment ==
  Input : Inport
  Demux : Demux
  Gain9 : Gain  Gain=S_w/2*b*Cl_f
  Product6 : Product
  Product7 : Product
  Sum7 : Sum  Inputs=|+-
  Out1 : Outport
  wires:
  Sum7/1 -> Gain9/1
  Product7/1 -> Sum7/2
  Product6/1 -> Sum7/1
  Gain9/1 -> Out1/1
  Demux/4 -> Product7/2
  Input/1 -> Demux/1
  Demux/2 -> Product7/1
  Demux/1 -> Product6/1
  Demux/3 -> Product6/2

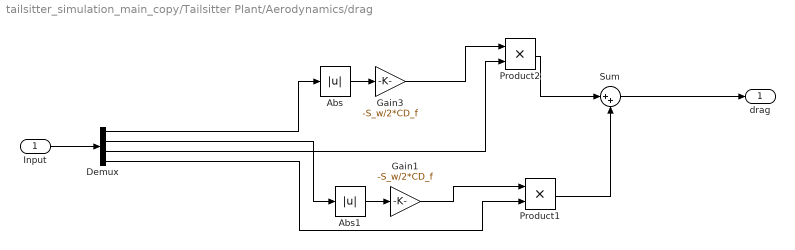
== system tailsitter_simulation_main_copy/Tailsitter Plant/Aerodynamics/drag ==
  Input : Inport
  Abs : Abs
  Abs1 : Abs
  Demux : Demux
  Gain1 : Gain  Gain=-S_w/2*CD_f
  Gain3 : Gain  Gain=-S_w/2*CD_f
  Product1 : Product
  Product2 : Product
  Sum : Sum  Inputs=|++
  drag : Outport
  wires:
  Demux/3 -> Product2/2
  Abs/1 -> Gain3/1
  Gain3/1 -> Product2/1
  Product2/1 -> Sum/1
  Demux/1 -> Abs/1
  Input/1 -> Demux/1
  Gain1/1 -> Product1/1
  Abs1/1 -> Gain1/1
  Demux/2 -> Abs1/1
  Demux/4 -> Product1/2
  Product1/1 -> Sum/2
  Sum/1 -> drag/1
